simulink model "MHIblock"  (R2014a)
settings: Solver=ode45  StartTime=0.0  StopTime=10.0  RelTol=1e-3
libraries: simulink x2
settings Model: CovSFcnEnable=on  Creator=student  LastModifiedBy=Jaromir
settings DataIOCC: SignalLoggingSaveFormat=ModelDataLogs
settings OptimizationCC: ExpressionDepthLimit=2147483647
settings DebuggingCC: UnderspecifiedInitializationDetection=Classic  FcnCallInpInsideContextMsg=UseLocalSettings  FrameProcessingCompatibilityMsg=error  StateNameClashWarn=warning  StrictBusMsg=Warning
settings GRTTargetCC: CombineOutputUpdateFcns=off  GRTInterface=on

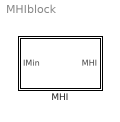
== system MHIblock ==
  MHI : Subsystem  mask{tres=12, Tau=6}
      mask prompts: tres "Motion treshold"; Tau "Tau parameter"

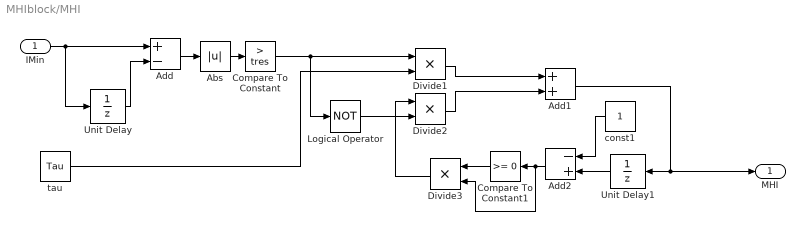
== system MHIblock/MHI ==
  IMin : Inport
  Abs : Abs
  Add : Sum  Inputs=+-  OutDataTypeStr=int16
  Add1 : Sum  OutDataTypeStr=double
  Add2 : Sum  Inputs=-+  OutDataTypeStr=double
  Compare To Constant : simulink/Logic and Bit Operations/Compare To Constant  relop=>  const=tres  OutDataTypeStr=uint8  ZeroCross=off
  Compare To Constant1 : simulink/Logic and Bit Operations/Compare To Constant  relop=>=  const=0  OutDataTypeStr=uint8  ZeroCross=off
  Divide1 : Product  Inputs=**
  Divide2 : Product  Inputs=**
  Divide3 : Product  Inputs=**
  Logical Operator : Logic  Operator=NOT  AllPortsSameDT=off  OutDataTypeStr=boolean
  Unit Delay : UnitDelay  SampleTime=-1
  Unit Delay1 : UnitDelay  SampleTime=-1
  const1 : Constant
  tau : Constant  Value=Tau
  MHI : Outport
  wires:
  Unit Delay/1 -> Add/2
  Add/1 -> Abs/1
  Abs/1 -> Compare To Constant/1
  tau/1 -> Divide1/2
  Logical Operator/1 -> Divide2/2
  Divide1/1 -> Add1/1
  Divide2/1 -> Add1/2
  Add1/1 -> Unit Delay1/1, MHI/1
  Unit Delay1/1 -> Add2/2
  const1/1 -> Add2/1
  Add2/1 -> Compare To Constant1/1, Divide3/2
  Compare To Constant1/1 -> Divide3/1
  Divide3/1 -> Divide2/1
  IMin/1 -> Add/1, Unit Delay/1
  Compare To Constant/1 -> Logical Operator/1, Divide1/1
